simulink model "RBNN_NNT_NN_comparision_exp1_ZOHHH"  (R2019a)
settings: Solver=FixedStepAuto  StartTime=0.0  StopTime=inf  FixedStep=0.000001  RelTol=1e-3
libraries: dsparch4 x3, dspstat3 x2
settings Model: Creator=vardhah  LastModifiedBy=vardhah
settings SolverCC: ConcurrentTasks=on  AutoInsertRateTranBlk=on
settings DataIOCC: ReturnWorkspaceOutputs=off
settings DebuggingCC: UnderSpecifiedDimensionMsg=warning  ArithmeticOperatorsInVariantConditions=warning

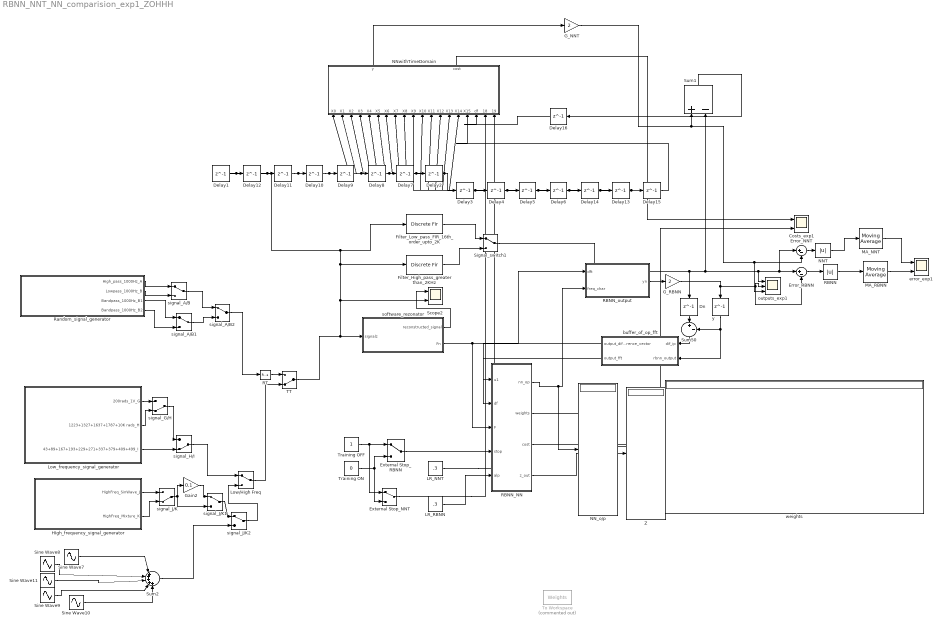
== system RBNN_NNT_NN_comparision_exp1_ZOHHH ==
  Costs_exp1 : Scope  NumInputPorts=2
  Delay{1..16} (16 alike) : Delay  DelayLength=1  InitialCondition=0
  Dn : Delay  DelayLength=1  InitialCondition=0
  Error_NNT : Sum  Inputs=|+-
  Error_RBNN : Sum  Inputs=|+-
  External Stop_NNT : ManualSwitch
  External Stop_RBNN : ManualSwitch
  Filter_High_pass_greater than_2KHz : DiscreteFir  Tag=BlockMethodSubSystem  Coefficients=[-0.0225862995506605629 -0.0314120930959356018 -0.0428930397338703126 -0.0586141314435711935 -0.0819989572139880191 -0.121996035222353263 -0.211508085226471271 -0.646964121963130134 0.646964121963130134 0.211508085226471271 0.121996035222353263 0.0819989572139880191 0.0586141314435711935 0.0428930397338703126 0.0314120930959356018 0.0225862995506605629]  InputProcessing=Columns as channels (frame based)
  Filter_Low_pass_FIR_16th_order_upto_2K : DiscreteFir  Tag=BlockMethodSubSystem  Coefficients=[-0.198889914644374777 0.0882189428518377339 0.0736891495871065116 0.0638368801789635787 0.0566372642221577294 0.0523172683654103132 0.0494565343907736044 0.048157521822162791 0.048157521822162791 0.0494565343907736044 0.0523172683654103132 0.0566372642221577294 0.0638368801789635787 0.0736891495871065116 0.0882189428518377339 -0.198889914644374777]  InputProcessing=Columns as channels (frame based)
  G_NNT : Gain  Gain=2
  G_RBNN : Gain  Gain=2
  Gain2 : Gain  Gain=0.1
  HIgh_frequency_signal_generator : Subsystem
  LR_NNT : Constant  Value=.3
  LR_RBNN : Constant  Value=.3
  Low/High Freq : ManualSwitch
  "Low_frequency_signal_generator " : Subsystem
  MA_NNT : dspstat3/Moving Average  Method=Sliding window  ForgettingFactorPort=off  SpecifyWindowLength=on  WindowLength=1  ForgettingFactor=0.9  SimulateUsing=Code generation
  MA_RBNN : dspstat3/Moving Average  Method=Sliding window  ForgettingFactorPort=off  SpecifyWindowLength=on  WindowLength=1  ForgettingFactor=0.9  SimulateUsing=Code generation
  NNT : Abs
  NN_o/p : Display
  NNwithTimeDomain : MATLAB Function  TreatAsAtomicUnit=on
  RBNN : Abs
  RBNN_NN : MATLAB Function  TreatAsAtomicUnit=on
  RBNN_output : MATLAB Function  TreatAsAtomicUnit=on
  RT : RateTransition  Deterministic=off  OutPortSampleTime=1e-06
  Random_signal_generator : Subsystem
  Scope2 : Scope  NumInputPorts=2
  Signal_switch1 : ManualSwitch
  Sine Wave10 : Sin  Amplitude=4  Frequency=58000  SampleTime=0
  Sine Wave11 : Sin  Amplitude=3  Frequency=33637  SampleTime=0
  Sine Wave7 : Sin  Amplitude=3  Frequency=58230  SampleTime=0
  Sine Wave8 : Sin  Amplitude=1.5  Frequency=37927  SampleTime=0
  Sine Wave9 : Sin  Amplitude=4  Frequency=59787  SampleTime=0
  Sum1 : Sum  Inputs=+-
  Sum2 : Sum  Inputs=|+++++
  Sum50 : Sum  Inputs=|+-
  TT : ManualSwitch  CurrentSetting=0
  To Workspace : ToWorkspace  Commented=on  VariableName=Weights  SaveFormat=Timeseries  SampleTime=-1
  Training OFF : Constant
  Training ON : Constant  Value=0
  Z : Display
  buffer_of_op_fft : MATLAB Function  TreatAsAtomicUnit=on
  error_exp1 : Scope  NumInputPorts=2
  outputs_exp1 : Scope  NumInputPorts=3
  signal_A/B : ManualSwitch
  signal_A/B1 : ManualSwitch
  signal_A/B2 : ManualSwitch
  signal_G/H : ManualSwitch  CurrentSetting=0
  signal_H/I : ManualSwitch  CurrentSetting=0
  signal_J/K : ManualSwitch  CurrentSetting=0
  signal_J/K1 : ManualSwitch
  signal_J/K2 : ManualSwitch
  software_rezonator : MATLAB Function  TreatAsAtomicUnit=on
  weights : Display
  y : Delay  DelayLength=1  InitialCondition=0
  wires:
  software_rezonator/1(reconstructed_signal) -> Scope2/1
  software_rezonator/2(Fn) -> RBNN_NN/3(F), RBNN_output/1(dft)
  Dn/1 -> Sum50/1
  y/1 -> buffer_of_op_fft/2(rbnn_output), Sum50/2
  RBNN_NN/1(nn_op) -> NN_o/p/1, RBNN_output/2(freq_char)
  External Stop_RBNN/1 -> RBNN_NN/4(stop)
  Training OFF/1 -> External Stop_NNT/1, External Stop_RBNN/1
  Training ON/1 -> External Stop_NNT/2, External Stop_RBNN/2
  RBNN_NN/3(cost) -> Costs_exp1/2
  RBNN_NN/2(weights) -> weights/1
  RBNN_NN/4(z_out) -> Z/1
  Sum50/1 -> buffer_of_op_fft/1(dif_ip)
  buffer_of_op_fft/1(output_difference_vector) -> RBNN_NN/2(df)
  buffer_of_op_fft/2(output_fft) -> RBNN_NN/1(u1)
  NNwithTimeDomain/1(y) -> G_NNT/1
  Delay16/1 -> NNwithTimeDomain/17(df)
  Delay4/1 -> NNwithTimeDomain/11(X10), Delay5/1
  Delay6/1 -> Delay14/1, NNwithTimeDomain/13(X12)
  Delay5/1 -> NNwithTimeDomain/12(X11), Delay6/1
  NNwithTimeDomain/2(cost) -> Costs_exp1/1
  Delay2/1 -> Delay3/1, NNwithTimeDomain/9(X8)
  Delay15/1 -> NNwithTimeDomain/16(X15)
  Delay13/1 -> Delay15/1, NNwithTimeDomain/15(X14)
  Delay14/1 -> Delay13/1, NNwithTimeDomain/14(X13)
  Delay10/1 -> NNwithTimeDomain/5(X4), Delay9/1
  TT/1 -> software_rezonator/1(signalz), Delay1/1, NNwithTimeDomain/1(X0), Filter_Low_pass_FIR_16th_order_upto_2K/1, Filter_High_pass_greater than_2KHz/1, Scope2/2
  Delay3/1 -> Delay4/1, NNwithTimeDomain/10(X9)
  Delay7/1 -> Delay2/1, NNwithTimeDomain/8(X7)
  Delay8/1 -> NNwithTimeDomain/7(X6), Delay7/1
  Delay1/1 -> NNwithTimeDomain/2(X1), Delay12/1
  Delay9/1 -> Delay8/1, NNwithTimeDomain/6(X5)
  Delay12/1 -> NNwithTimeDomain/3(X2), Delay11/1
  Delay11/1 -> Delay10/1, NNwithTimeDomain/4(X3)
  Sum1/1 -> Delay16/1
  Filter_High_pass_greater than_2KHz/1 -> Signal_switch1/2
  Filter_Low_pass_FIR_16th_order_upto_2K/1 -> Signal_switch1/1
  Signal_switch1/1 -> Dn/1, outputs_exp1/1, Error_NNT/1, Error_RBNN/1, Sum1/2
  Error_RBNN/1 -> RBNN/1
  Error_NNT/1 -> NNT/1
  G_NNT/1 -> outputs_exp1/3, Error_NNT/2, Sum1/1
  LR_RBNN/1 -> RBNN_NN/5(alp)
  RBNN/1 -> MA_RBNN/1
  Random_signal_generator/1(High_pass_1000Hz_A) -> signal_A/B/1
  Random_signal_generator/2(Lowpass_1000Hz_B) -> signal_A/B/2
  signal_G/H/1 -> signal_H/I/1
  Low/High Freq/1 -> TT/2
  NNT/1 -> MA_NNT/1
  MA_NNT/1 -> error_exp1/1
  MA_RBNN/1 -> error_exp1/2
  External Stop_NNT/1 -> NNwithTimeDomain/18(stop)
  RBNN_output/1(yn) -> G_RBNN/1
  "Low_frequency_signal_generator "/1(200rads_1V_G) -> signal_G/H/1
  "Low_frequency_signal_generator "/2(1223+1327+1637+1787+10K rads_H) -> signal_G/H/2
  "Low_frequency_signal_generator "/3(43+89+167+193+229+271+337+379+409+499_I) -> signal_H/I/2
  HIgh_frequency_signal_generator/1(HighFreq_SinWave_J) -> signal_J/K/1
  HIgh_frequency_signal_generator/2(HighFreq_Mixture_K) -> signal_J/K/2
  signal_J/K/1 -> signal_J/K1/2, Gain2/1
  signal_H/I/1 -> Low/High Freq/1
  Gain2/1 -> signal_J/K1/1
  LR_NNT/1 -> NNwithTimeDomain/19(alpha_l)
  Sine Wave11/1 -> Sum2/3
  Sine Wave10/1 -> Sum2/5
  Sine Wave8/1 -> Sum2/2
  Sine Wave9/1 -> Sum2/4
  Sum2/1 -> signal_J/K2/2
  Sine Wave7/1 -> Sum2/1
  signal_J/K1/1 -> signal_J/K2/1
  signal_J/K2/1 -> Low/High Freq/2
  G_RBNN/1 -> y/1, outputs_exp1/2, Error_RBNN/2
  signal_A/B/1 -> signal_A/B2/1
  Random_signal_generator/3(Bandpass_1000Hz_B1) -> signal_A/B1/1
  signal_A/B2/1 -> RT/1
  Random_signal_generator/4(Bandpass_1000Hz_B2) -> signal_A/B1/2
  signal_A/B1/1 -> signal_A/B2/2
  RT/1 -> TT/1

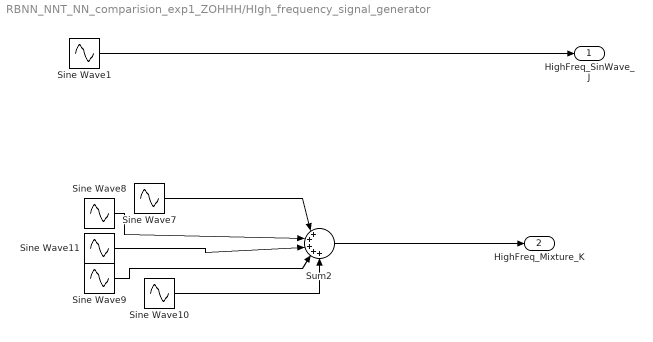
== system RBNN_NNT_NN_comparision_exp1_ZOHHH/HIgh_frequency_signal_generator ==
  Sine Wave1 : Sin  Amplitude=3  Frequency=50000  SampleTime=0
  Sine Wave10 : Sin  Amplitude=2  Frequency=47000  SampleTime=0
  Sine Wave11 : Sin  Amplitude=2  Frequency=30637  SampleTime=0
  Sine Wave7 : Sin  Amplitude=2  Frequency=28230  SampleTime=0
  Sine Wave8 : Sin  Amplitude=2  Frequency=33927  SampleTime=0
  Sine Wave9 : Sin  Amplitude=2  Frequency=53787  SampleTime=0
  Sum2 : Sum  Inputs=|+++++
  HighFreq_SinWave_J : Outport
  HighFreq_Mixture_K : Outport  Port=2
  wires:
  Sine Wave9/1 -> Sum2/4
  Sum2/1 -> HighFreq_Mixture_K/1
  Sine Wave7/1 -> Sum2/1
  Sine Wave10/1 -> Sum2/5
  Sine Wave8/1 -> Sum2/2
  Sine Wave1/1 -> HighFreq_SinWave_J/1
  Sine Wave11/1 -> Sum2/3

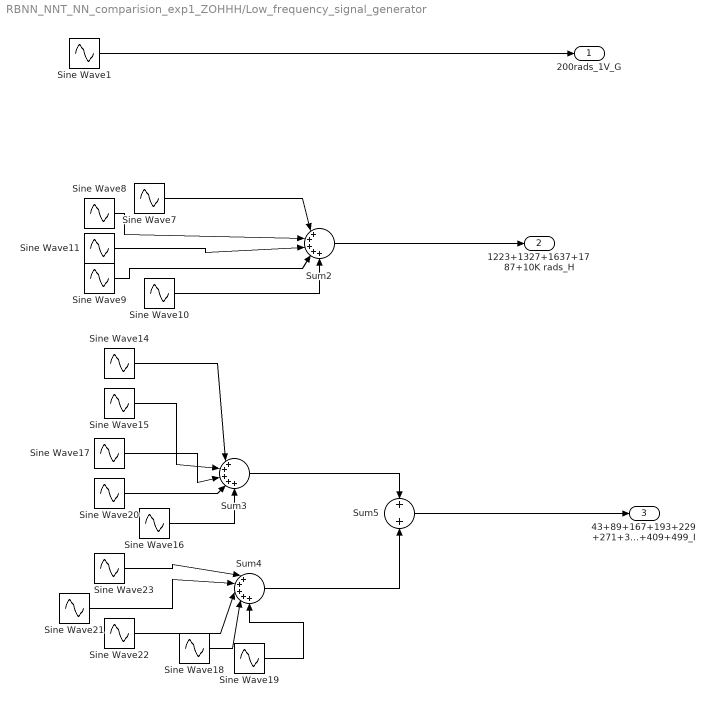
== system RBNN_NNT_NN_comparision_exp1_ZOHHH/Low_frequency_signal_generator  ==
  Sine Wave1 : Sin  Amplitude=0.9  Frequency=200  SampleTime=0
  Sine Wave10 : Sin  Amplitude=0.2  Frequency=10000  SampleTime=0
  Sine Wave11 : Sin  Amplitude=0.2  Frequency=1637  SampleTime=0
  Sine Wave14 : Sin  Amplitude=0.05  Frequency=43  SampleTime=0
  Sine Wave15 : Sin  Amplitude=0.1  Frequency=89  SampleTime=0
  Sine Wave16 : Sin  Amplitude=0.1  Frequency=229  SampleTime=0
  Sine Wave17 : Sin  Amplitude=0.1  Frequency=167  SampleTime=0
  Sine Wave18 : Sin  Amplitude=0.1  Frequency=409  SampleTime=0
  Sine Wave19 : Sin  Amplitude=0.1  Frequency=499  SampleTime=0
  Sine Wave20 : Sin  Amplitude=0.1  Frequency=193  SampleTime=0
  Sine Wave21 : Sin  Amplitude=0.1  Frequency=337  SampleTime=0
  Sine Wave22 : Sin  Amplitude=0.1  Frequency=379  SampleTime=0
  Sine Wave23 : Sin  Amplitude=0.05  Frequency=271  SampleTime=0
  Sine Wave7 : Sin  Amplitude=0.1  Frequency=1223  SampleTime=0
  Sine Wave8 : Sin  Amplitude=0.2  Frequency=1327  SampleTime=0
  Sine Wave9 : Sin  Amplitude=0.2  Frequency=1787  SampleTime=0
  Sum2 : Sum  Inputs=|+++++
  Sum3 : Sum  Inputs=|+++++
  Sum4 : Sum  Inputs=|+++++
  Sum5 : Sum
  200rads_1V_G : Outport
  1223+1327+1637+1787+10K rads_H : Outport  Port=2
  43+89+167+193+229+271+337+379+409+499_I : Outport  Port=3
  wires:
  Sine Wave7/1 -> Sum2/1
  Sine Wave8/1 -> Sum2/2
  Sine Wave11/1 -> Sum2/3
  Sine Wave9/1 -> Sum2/4
  Sine Wave10/1 -> Sum2/5
  Sum3/1 -> Sum5/1
  Sum4/1 -> Sum5/2
  Sine Wave14/1 -> Sum3/1
  Sine Wave19/1 -> Sum4/5
  Sine Wave21/1 -> Sum4/2
  Sine Wave16/1 -> Sum3/5
  Sine Wave15/1 -> Sum3/2
  Sine Wave17/1 -> Sum3/3
  Sine Wave20/1 -> Sum3/4
  Sine Wave23/1 -> Sum4/1
  Sine Wave18/1 -> Sum4/4
  Sine Wave22/1 -> Sum4/3
  Sum5/1 -> 43+89+167+193+229+271+337+379+409+499_I/1
  Sine Wave1/1 -> 200rads_1V_G/1
  Sum2/1 -> 1223+1327+1637+1787+10K rads_H/1

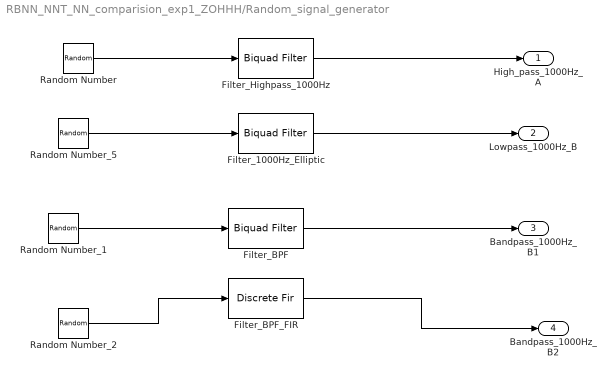
== system RBNN_NNT_NN_comparision_exp1_ZOHHH/Random_signal_generator ==
  Filter_1000Hz_Elliptic : dsparch4/Biquad Filter  Tag=BlockMethodSubSystem  FilterSource=Dialog parameters  CoeffSource=Specify via dialog  FilterObject=BQF  IIRFiltStruct=Direct form II  BiQuadCoeffs=[1 -1.97632274641133088 1 1 -1.97939835930391728 0.996447647782941925;1 -1.97278944538463175 1 1 -1.97237302925889701 0.987301248342435933;1 -1.95955871016892758 1 1 -1.96235771308246942 0.972660421241710926;1 -1.88453112329299022 1 1 -1.95007892273323602 0.954154972801176005;1 1 0 1 -0.971866907997287366 0]  ScaleValues=[0.156742012624585314;0.548618699418480849;0.254757160374388947;0.035299988916345823;0.064621492680459483;1]  IC=0  ICnum=0  ICden=0  a0Flag=Warning  optimizeScaleValues=on  ScaleValueMode=Specify via input port (g)  InputProcessing=Columns as channels (frame based)  roundingMode=Floor  overflowMode=off  scaleValueFracLength=14  denProdOutputFracLength=30  denAccumFracLength=30  secondMemoryFracLength=15
      settings: SourceProductName=DSP System Toolbox
  Filter_BPF : dsparch4/Biquad Filter  Tag=BlockMethodSubSystem  FilterSource=Dialog parameters  CoeffSource=Specify via dialog  FilterObject=BQF  IIRFiltStruct=Direct form II  BiQuadCoeffs=[1 1.34543140640054615 1 1 -0.865836953112267715 0.912596166370734707;1 -1.20629005563207525 1 1 1.0374782377076639 0.917360750285181492;1 1.40379640773364511 1 1 0.956203030482965288 0.761149491110006959;1 -1.2743706631397218 1 1 -0.795182822059391725 0.748508882192643776;1 1.52447215639555766 1 1 0.866143741073349682 0.602125300492039273;1 -1.41675424185331345 1 1 -0.715853042247783122 0.583156859691732254;1 1.70522262642585898 1 1 0.737950084029138531 0.429992816928946642;1 -1.63419928080231425 1 1 -0.597519721319533126 0.407141060566249324;1 1.90382856695961999 1 1 0.517283407442173937 0.245793186973016303;1 -1.87909567943918843 1 1 -0.384060965389813713 0.225520142949825281;1 0 -1 1 0.065271972301287659 0.111238951995475455]  ScaleValues=[0.748980110690750434;0.748980110690750434;0.679045523645565474;0.679045523645565474;0.604852900866532095;0.604852900866532095;0.530110720433375038;0.530110720433375038;0.469038099590365576;0.469038099590365576;0.4443805240022623;1]  IC=0  ICnum=0  ICden=0  a0Flag=Warning  optimizeScaleValues=on  ScaleValueMode=Specify via input port (g)  InputProcessing=Columns as channels (frame based)  roundingMode=Floor  overflowMode=off  scaleValueFracLength=14  denProdOutputFracLength=30  denAccumFracLength=30  secondMemoryFracLength=15
      settings: SourceProductName=DSP System Toolbox
  Filter_BPF_FIR : DiscreteFir  Tag=BlockMethodSubSystem  Coefficients=[0.000405311015767818416 -0.000340162424744905724 -0.00275017457650896012 -0.00174274245080286837 0.00514491904143095716 0.00647577832444998051 -0.00568854990170439972 -0.0126842654631062011 0.00248179604874338095 0.0160107744241187906 0.00223850273897984765 -0.0125757061527468211 -0.00141279599705250057 0.00406157889441875145 -0.0126642406219731191 -1.85837801898820644e-05 0.0408268777064352897 0.0133647214892564613 -0.0722859420326916191 -0.0505173101841354111 0.0883091271404974482 0.103364573239606156 -0.0737806038715707602 -0.150637807286995051 0.0288308946921712328 0.169635266121260897 0.0288308946921712328 -0.150637807286995051 -0.0737806038715707602 0.103364573239606156 0.0883091271404974482 -0.0505173101841354111 -0.0722859420326916191 0.0133647214892564613 0.0408268777064352897 -1.85837801898820644e-05 -0.0126642406219731191 0.00406157889441875145 -0.00141279599705250057 -0.0125757061527468211 0.00223850273897984765 0.0160107744241187906 0.00248179604874338095 -0.0126842654631062011 -0.00568854990170439972 0.00647577832444998051 0.00514491904143095716 -0.00174274245080286837 -0.00275017457650896012 -0.000340162424744905724 0.000405311015767818416]  InputProcessing=Columns as channels (frame based)
  Filter_Highpass_1000Hz : dsparch4/Biquad Filter  Tag=BlockMethodSubSystem  FilterSource=Dialog parameters  CoeffSource=Specify via dialog  FilterObject=BQF  IIRFiltStruct=Direct form II  BiQuadCoeffs=[1 -1.9832348135082305 1 1 -1.92871230100246671 0.962722433368264241;1 -1.98583197848424597 1 1 -1.86448430214602556 0.894880266245439038;1 -1.99020937824944788 1 1 -1.81348943480495617 0.839000119522318677;1 -1.99498360843622446 1 1 -1.77690733715439997 0.797591087467987903;1 -1.99863653257112794 1 1 -1.75501257669195576 0.772196386514157451;1 -1 0 1 -0.873867637211059756 0]  ScaleValues=[0.976953385016072651;0.943181897451958351;0.915362881516173843;0.894746706112661938;0.882102920451765637;0.936933818605529933;1]  IC=0  ICnum=0  ICden=0  a0Flag=Warning  optimizeScaleValues=on  ScaleValueMode=Specify via input port (g)  InputProcessing=Columns as channels (frame based)  roundingMode=Floor  overflowMode=off  scaleValueFracLength=14  denProdOutputFracLength=30  denAccumFracLength=30  secondMemoryFracLength=15
      settings: SourceProductName=DSP System Toolbox
  Random Number : RandomNumber  Variance=0.2  SampleTime=0.00001
  Random Number_1 : RandomNumber  Mean=0.1  Variance=0.4  SampleTime=0.00002
  Random Number_2 : RandomNumber  Variance=0.5  SampleTime=0.00001
  Random Number_5 : RandomNumber  Variance=0.5  SampleTime=0.00001
  High_pass_1000Hz_A : Outport
  Lowpass_1000Hz_B : Outport  Port=2
  Bandpass_1000Hz_B1 : Outport  Port=3
  Bandpass_1000Hz_B2 : Outport  Port=4
  wires:
  Random Number/1 -> Filter_Highpass_1000Hz/1
  Filter_Highpass_1000Hz/1 -> High_pass_1000Hz_A/1
  Random Number_5/1 -> Filter_1000Hz_Elliptic/1
  Filter_1000Hz_Elliptic/1 -> Lowpass_1000Hz_B/1
  Random Number_1/1 -> Filter_BPF/1
  Filter_BPF/1 -> Bandpass_1000Hz_B1/1
  Random Number_2/1 -> Filter_BPF_FIR/1
  Filter_BPF_FIR/1 -> Bandpass_1000Hz_B2/1

== matlab function RBNN_NNT_NN_comparision_exp1_ZOHHH/RBNN_NN ==
  settings: sampleTime=0.01
  data: u1 input size=[1,16]; df input size=[1,16]; F input size=16; nn_op output size=16; weights output; cost output; z_out output; stop input; alp input
function [nn_op,weights,cost,z_out]  = NN(u1,df,F,stop,alp)

persistent w1;
persistent vy;
persistent g;
persistent itr;
persistent J;
persistent del_w;
persistent mult;
persistent memory_alloc_flag;
persistent n; 

if isempty(n)
        n = 0; 
end
n=n+1; 

u2=1; 
alpha = alp;
%layer declaration
input_layer = 17; 
layer_1=16;

if isempty(memory_alloc_flag)
        memory_alloc_flag = 0; 
end
if isempty(mult)
       mult=zeros(layer_1,layer_1*input_layer); 
end
if memory_alloc_flag==0
 %write memory allocation for looped code here.. 
 mult=[];
  for itr =1:layer_1
   mult=[mult;[zeros(1,(itr-1)*input_layer) ones(1,input_layer) zeros(1,(input_layer-itr-1)*input_layer)]];
 end
 memory_alloc_flag=1;
end

if isempty(del_w)
    del_w=zeros(1,272);
end

if isempty(itr)
    itr=0;
end
if isempty(J)
    J=0;
end

%gradient initialisation
if isempty(g)
    g= zeros(16,272);
   %g= rand(16,272);   
end


%prestored Vy matrix
if isempty(vy)
    vy=[0.0625000000000000,0.0625000000000000,0.0625000000000000,0.0625000000000000,0.0625000000000000,0.0625000000000000,0.0625000000000000,0.0625000000000000,0.0625000000000000,0.0625000000000000,0.0625000000000000,0.0625000000000000,0.0625000000000000,0.0625000000000000,0.0625000000000000,0.0625000000000000;0.0577424707819554,0.0441941738241592,0.0239177145228181,-1.14810637420064e-17,-0.0239177145228181,-0.0441941738241592,-0.0577424707819554,-0.0625000000000000,-0.0577424707819554,-0.0441941738241592,-0.0239177145228181,3.82702124733548e-18,0.0239177145228181,0.0441941738241592,0.0577424707819554,0.0625000000000000;0.0441941738241592,-2.67891487313484e-17,-0.0441941738241592,-0.0625000000000000,-0.0441941738241592,1.91351062366774e-17,0.0441941738241592,0.0625000000000000,0.0441941738241592,-1.14810637420064e-17,-0.0441941738241592,-0.0625000000000000,-0.0441941738241592,3.82702124733548e-18,0.0441941738241592,0.0625000000000000;0.0239177145228179,-0.0441941738241592,-0.0577424707819554,3.44431912260193e-17,0.0577424707819555,0.0441941738241592,-0.0239177145228182,-0.0625000000000000,-0.0239177145228181,0.0441941738241592,0.0577424707819554,-1.14810637420064e-17,-0.0577424707819554,-0.0441941738241592,0.0239177145228181,0.0625000000000000;-1.68427621172548e-16,-0.0625000000000000,-6.12710262471544e-17,0.0625000000000000,-1.53119536183206e-16,-0.0625000000000000,3.44431912260193e-17,0.0625000000000000,-2.67891487313484e-17,-0.0625000000000000,1.91351062366774e-17,0.0625000000000000,-1.14810637420064e-17,-0.0625000000000000,3.82702124733548e-18,0.0625000000000000;-0.0239177145228182,-0.0441941738241591,0.0577424707819554,-1.68427621172548e-16,-0.0577424707819554,0.0441941738241592,0.0239177145228181,-0.0625000000000000,0.0239177145228182,0.0441941738241592,-0.0577424707819554,1.91351062366774e-17,0.0577424707819554,-0.0441941738241592,-0.0239177145228181,0.0625000000000000;-0.0441941738241596,-3.06548562684706e-17,0.0441941738241593,-0.0625000000000000,0.0441941738241594,-1.68427621172548e-16,-0.0441941738241592,0.0625000000000000,-0.0441941738241592,3.44431912260193e-17,0.0441941738241592,-0.0625000000000000,0.0441941738241592,-1.14810637420064e-17,-0.0441941738241592,0.0625000000000000;-0.0577424707819556,0.0441941738241594,-0.0239177145228178,-3.06548562684706e-17,0.0239177145228179,-0.0441941738241591,0.0577424707819554,-0.0625000000000000,0.0577424707819555,-0.0441941738241592,0.0239177145228182,-2.67891487313484e-17,-0.0239177145228181,0.0441941738241592,-0.0577424707819554,0.0625000000000000;-0.0625000000000000,0.0625000000000000,-0.0625000000000000,0.0625000000000000,-0.0625000000000000,0.0625000000000000,-0.0625000000000000,0.0625000000000000,-0.0625000000000000,0.0625000000000000,-0.0625000000000000,0.0625000000000000,-0.0625000000000000,0.0625000000000000,-0.0625000000000000,0.0625000000000000;-0.0239177145228184,0.0441941738241592,-0.0577424707819555,0.0625000000000000,-0.0577424707819553,0.0441941738241592,-0.0239177145228180,-6.88863824520386e-17,0.0239177145228181,-0.0441941738241593,0.0577424707819554,-0.0625000000000000,0.0577424707819554,-0.0441941738241592,0.0239177145228181,0;-0.0441941738241594,0.0625000000000000,-0.0441941738241593,-3.36855242345096e-16,0.0441941738241595,-0.0625000000000000,0.0441941738241592,7.65404249467096e-17,-0.0441941738241593,0.0625000000000000,-0.0441941738241592,-3.82702124733548e-17,0.0441941738241593,-0.0625000000000000,0.0441941738241592,0;-0.0577424707819556,0.0441941738241592,0.0239177145228178,-0.0625000000000000,0.0239177145228177,0.0441941738241592,-0.0577424707819555,-3.06239072366412e-16,0.0577424707819554,-0.0441941738241592,-0.0239177145228181,0.0625000000000000,-0.0239177145228181,-0.0441941738241593,0.0577424707819554,0;-0.0625000000000000,6.13097125369412e-17,0.0625000000000000,1.37772764904077e-16,-0.0625000000000000,-3.36855242345096e-16,0.0625000000000000,9.18485099360515e-17,-0.0625000000000000,-6.88863824520386e-17,0.0625000000000000,4.59242549680257e-17,-0.0625000000000000,-2.29621274840129e-17,0.0625000000000000,0;-0.0577424707819553,-0.0441941738241594,0.0239177145228181,0.0625000000000000,0.0239177145228186,-0.0441941738241590,-0.0577424707819555,1.22542052494309e-16,0.0577424707819554,0.0441941738241593,-0.0239177145228180,-0.0625000000000000,-0.0239177145228182,0.0441941738241592,0.0577424707819554,0;-0.0441941738241587,-0.0625000000000000,-0.0441941738241588,6.13097125369412e-17,0.0441941738241588,0.0625000000000000,0.0441941738241592,1.07156594925393e-16,-0.0441941738241590,-0.0625000000000000,-0.0441941738241593,-5.35782974626967e-17,0.0441941738241592,0.0625000000000000,0.0441941738241592,0;-0.0239177145228178,-0.0441941738241593,-0.0577424707819556,-0.0625000000000000,-0.0577424707819556,-0.0441941738241594,-0.0239177145228184,-3.36855242345096e-16,0.0239177145228181,0.0441941738241592,0.0577424707819554,0.0625000000000000,0.0577424707819554,0.0441941738241593,0.0239177145228182,0;0,0,0,0,0,0,0,0,0,0,0,0,0,0,0,0];
end



%input initialisation
x_in = [real(u1(1)) real(u1(2)) real(u1(3)) real(u1(4)) real(u1(5)) real(u1(6)) real(u1(7)) real(u1(8)) real(u1(9)) imag(u1(1)) imag(u1(2)) imag(u1(3)) imag(u1(4)) imag(u1(5)) imag(u1(6)) imag(u1(7))];

%parameter intialisation 
v=transpose([x_in u2]);
if isempty(w1)
       w1=randn(input_layer,layer_1)*0.1;
end


%F=transpose([real(X0) 2*(real(X1)*cos(pi*1*n/8)-imag(X1)*sin(pi*1*n/8)) 2*(real(X2)*cos(pi*2*n/8)-imag(X2)*sin(pi*2*n/8)) 2*(real(X3)*cos(pi*3*n/8)-imag(X3)*sin(pi*3*n/8)) 2*(real(X4)*cos(pi*4*n/8)-imag(X4)*sin(pi*4*n/8)) 2*(real(X5)*cos(pi*5*n/8)-imag(X5)*sin(pi*5*n/8)) 2*(real(X6)*cos(pi*6*n/8)-imag(X6)*sin(pi*6*n/8)) 2*(real(X7)*cos(pi*7*n/8)-imag(X7)*sin(pi*7*n/8)) -1^n*real(X8) -2*(imag(X9)*cos(pi*9*n/8)+real(X9)*sin(pi*9*n/8)) -2*(imag(X10)*cos(pi*10*n/8)+real(X10)*sin(pi*10*n/8)) -2*(imag(X11)*cos(pi*11*n/8)+real(X11)*sin(pi*11*n/8)) -2*(imag(X12)*cos(pi*12*n/8)+real(X12)*sin(pi*12*n/8)) -2*(imag(X13)*cos(pi*13*n/8)+real(X13)*sin(pi*13*n/8)) -2*(imag(X14)*cos(pi*14*n/8)+real(X14)*sin(pi*14*n/8)) -2*(imag(X15)*cos(pi*15*n/8)+real(X15)*sin(pi*15*n/8))]); 
%u_out=v;


%forward propogation
z=w1'*v ;
z_out=z;
a=(1./(1+exp(-z)));
an=(a-0.5);

%calculation of Nv:
dz_a=a.*(1-a);                  
Nv=w1'.* repmat(dz_a,1, size(w1,1));

%calculation of aD
aD=transpose(F)*Nv*vy;
A=[aD;eye(15) zeros(15,1)];
B=[transpose(F) ; zeros(15,16)];   
dw1=v*transpose(dz_a);

%added to vectorise the implementation
Expanded_dw1=repmat(transpose(dw1),1,size(dw1,2));
Nw=Expanded_dw1.*mult; 
g=A*g+B*Nw;



if mod(n,16)==0 && stop==0
    del_w =alpha*df*1*g/16 ;
    del_w_reshaped= reshape(del_w,[17,16]);
    w1=w1+ del_w_reshaped;
    itr=itr+1;
    
end

J= 1/2*df(1)^2;
cost=J;
weights=w1;


nn_op=an;


end

== matlab function RBNN_NNT_NN_comparision_exp1_ZOHHH/buffer_of_op_fft ==
  data: output_difference_vector output size=[1,16]; output_fft output size=[1,16]; dif_ip input; rbnn_output input
function [output_difference_vector,output_fft] = difBuffer(dif_ip,rbnn_output)                      

 sz=16;                       % size of the dft 
 
 persistent a;
 persistent b;
 if isempty(b)
  b= zeros(1,sz);
 end
 if isempty(a)
  a= zeros(1,sz);
 end
 
 
  a= circshift(a,1);
  a(1)=dif_ip;
  b= circshift(b,1);
  b(1)=rbnn_output;

 output_difference_vector=a; 
 output_fft=1/sz*fft(b); 
end

== matlab function RBNN_NNT_NN_comparision_exp1_ZOHHH/NNwithTimeDomain ==
  settings: sampleTime=0.125
  data: X0 input; X1 input; X2 input; X3 input; X4 input; X5 input; X6 input; X7 input; X8 input; X9 input; X10 input; X11 input; X12 input; X13 input; X14 input; X15 input; df input; y output; cost output; stop input; alpha_l input
function [y,cost] = NN(X0,X1,X2,X3,X4,X5,X6,X7,X8,X9,X10,X11,X12,X13,X14,X15,df,stop,alpha_l)

%This is a generalised code for 2 layer - multiple input-single output network.
% to alter the network (1) "change layer's size" in layer declaration below (2) the function
%input and output above and (3) Input matrix creation. (4) change inputs in
%simulink design

alpha = alpha_l;

%(1)layer decalration
layer_0= 16;
layer_1= 16;
layer_2 =1;


%(2) is above in function block

%(3)parameter intialisation
v=[X0 X1 X2 X3 X4 X5 X6 X7 X8 X9 X10 X11 X12 X13 X14 X15];

%Do not alter the code below. The below implementaion is generalised for
%multiple input and single output, 2 layer neural network. 


persistent w1 w2;
persistent a1 a2;
persistent J; 
persistent v_old; 

if isempty(a1)
    a1= zeros(layer_1,1);
end

if isempty(a2)
    a2= zeros(layer_2,1);
end


if isempty(J)
    J= 0;
end
if isempty(v_old)
    v_old= zeros(1,layer_0);
end



if isempty(w1)
       w1=randn(layer_1,layer_0);
end
if isempty(w2)
       w2=randn(layer_2,layer_1);
end

%BackProp:
if stop==0
dz2=a2.*(1-a2)*df*-1;
dw2=dz2*transpose(a1);
dz1=(a1.*(1-a1)).*(w2'*dz2);
%dz1=a1.*(1-a1)*dz2;
dw1=dz1*v;
w2=w2 + alpha*dw2;
w1=w1 + alpha*dw1;
v_old=v;
end 

%forward propogation
z1=w1*v';
a1= (1./(1+exp(-z1)));
an1=a1-0.5;
z2=w2*an1;
a2= (1./(1+exp(-z2)));
an2=a2-0.5;
cost=1/2*df^2;

%output assignment
y=an2;


end

== matlab function RBNN_NNT_NN_comparision_exp1_ZOHHH/software_rezonator ==
  data: signalz input; reconstructed_signal output size=1; Fn output size=16
function [reconstructed_signal,Fn]   = rezonator(signalz)

persistent numberofrezonator;
persistent g c bfr_rezo_sm aft_delay dft_out;
persistent out signal_dif;
persistent n;
persistent memory_alloc_flag;


%assign the number of rezonator here. For configuring it for higher order
%rezonator  we need to change (1) 'numberofrezonaotor' variable
if isempty(numberofrezonator)
        numberofrezonator = 16;   %here 16 parallel rezonators
end

%Initialisation of memory allocations/variables ====> 
if isempty(memory_alloc_flag)
        memory_alloc_flag = 0; 
end
if isempty(g)
       g=zeros(numberofrezonator,numberofrezonator,'like',0i); 
end
if isempty(c)
       c=zeros(numberofrezonator,numberofrezonator,'like',0i); 
end
if memory_alloc_flag==0
 for i=0:numberofrezonator-1
  for j= 0:numberofrezonator-1
   g(i+1,j+1)=1/numberofrezonator*(exp(-1i*2*pi*i*j/numberofrezonator));
   c(i+1,j+1)=(exp(1i*2*pi*i*j/numberofrezonator));
  end 
 end
 memory_alloc_flag=1;
end


%Initialisation of variables  =====> 
if isempty(n)
        n = 0;   
end 
if isempty(out)
  out=0+0i;
end
if isempty(signal_dif)
  signal_dif=0+0i;
end
if isempty(bfr_rezo_sm)
  bfr_rezo_sm=repmat(0+0i,numberofrezonator,1);
end
if isempty(aft_delay)
  aft_delay=repmat(0+0i,numberofrezonator,1);
end
if isempty(dft_out)
  dft_out=repmat(0+0i,numberofrezonator,1);
end

%creating cycle of rotation for selection of correct column of g & c.
cycle=mod(n,numberofrezonator);

%resonator core -----------------------------> 
dft_out=c(:,cycle+1).*aft_delay;
out= sum(dft_out,1);
signal_dif=signalz-out;
bfr_rezo_sm=g(:,cycle+1).*signal_dif;

%counting the counter
n=n+1;

% output assignment ------------------>
reconstructed_signal=out;
dft=aft_delay; 
N=16;
a=1:1:N/2-1;
b=N/2+1:1:N-1;
dft_trans=transpose(dft);
Fn=transpose([real(dft_trans(1)) 2*(real(dft_trans(2:N/2)).*cos(2*pi*a*n/N)-imag(dft_trans(2:N/2)).*sin(2*pi*a*n/N)) -1^n*real(dft_trans(N/2+1)) -2*(imag(dft_trans(N/2+2:N)).*cos(2*pi*b*n/N)+real(dft_trans(N/2+2:N)).*sin(2*pi*b*n/N))]);
%--------output assignment over----------<

%final updation of buffer ------>>>>>>>>>>>>
aft_delay= aft_delay+bfr_rezo_sm; 
end

== matlab function RBNN_NNT_NN_comparision_exp1_ZOHHH/RBNN_output ==
  data: dft input size=16; yn output size=1; freq_char input size=16
function yn = fcn(dft,freq_char)
yn=transpose(freq_char)*dft;
end
